simulink model "flightControlSystem"  (R2019a)
settings: Solver=ode3  StartTime=0  StopTime=TFinal  FixedStep=Ts  RelTol=1e-3  EnableMultiTasking=on
undefined symbols (not defined in the file): codertarget, Controller, DiscIntNeverNeededParam, Discrete, Estimator, g, I_pr_antiWU, I_pr_satLimitHigh, I_pr_satLimitLow, I_xy_antiWU, I_xy_satLimitHigh, I_xy_satLimitLow, I_z_antiWU, I_z_satLimitHigh, I_z_satLimitLow, init, Sensors, Time, Ts, Vehicle
libraries: simulink x35, sharedtransform x3, ctrlSharedLib x2, parrotlib x2, dspsigops x1, sharedutil x1
(part 1 of 2)

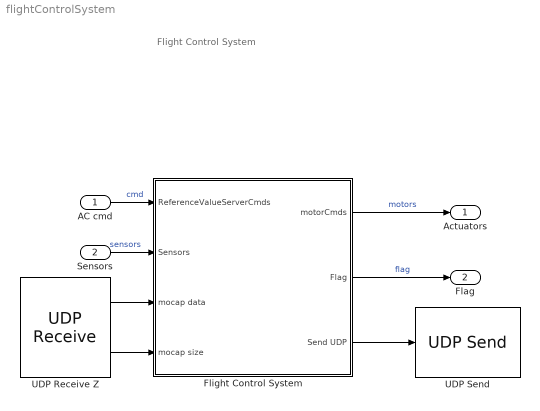
== system flightControlSystem ==
  note: Flight Control System
  AC cmd : Inport  OutDataTypeStr=Bus: CommandBus  BusOutputAsStruct=on
  Sensors : Inport  Port=2  OutDataTypeStr=Bus: SensorsBus  BusOutputAsStruct=on
  Flight Control System : Subsystem  InitFcn=codertarget.parrot.internal.fcsSubsystemCallback(gcb);  TreatAsAtomicUnit=on  SystemSampleTime=Ts
  UDP Receive Z : parrotlib/UDP Receive  localURL='0.0.0.0'  localPort=25000  remoteURL='0.0.0.0'  remotePort=-1  recvBufferSize=8192  signalDatatype=single  dims=24  isVarSize=off  showBlockingTime=off  blockingTime=0  sampletime=0.005  blockPlatform=LINUX
  UDP Send : parrotlib/UDP Send  remoteURL='192.168.3.2'  remotePort=25001  localURL='0.0.0.0'  localPortSource=Automatically determine  localPort=2048  sampletime=-1  blockPlatform=LINUX  separateLengthPort=0
  Actuators : Outport  OutDataTypeStr=single  PortDimensions=4
  Flag : Outport  Port=2  OutDataTypeStr=uint8  PortDimensions=1
  wires:
  Flight Control System/1(motorCmds) -> Actuators/1  "motors"
  Flight Control System/2(Flag) -> Flag/1  "flag"
  Flight Control System/3(Send UDP) -> UDP Send/1
  AC cmd/1 -> Flight Control System/1(ReferenceValueServerCmds)  "cmd"
  Sensors/1 -> Flight Control System/2(Sensors)  "sensors"
  UDP Receive Z/1 -> Flight Control System/3(mocap data)
  UDP Receive Z/2 -> Flight Control System/4(mocap size)

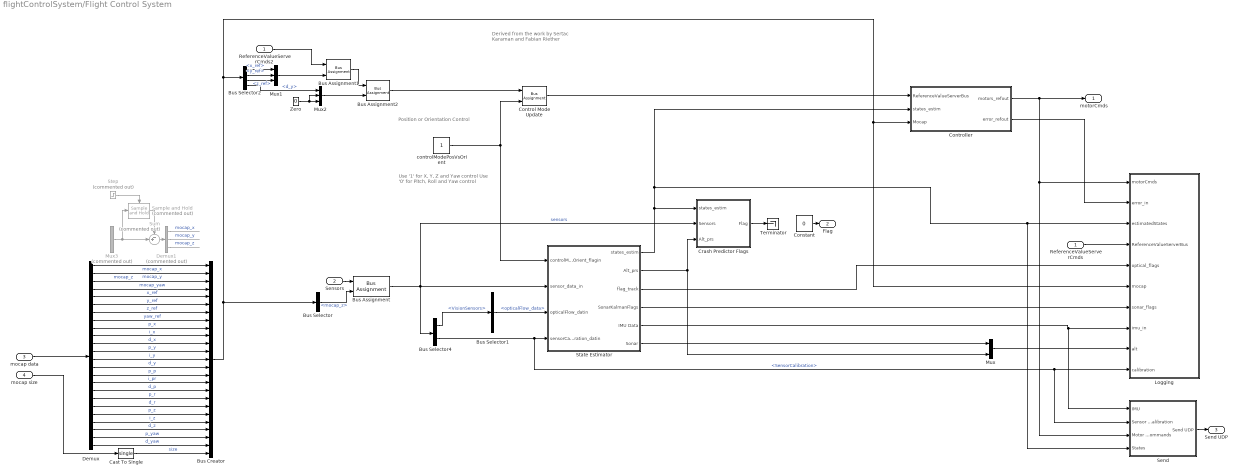
== system flightControlSystem/Flight Control System ==
  note: Use '1' for X, Y, Z and Yaw control
      | Use '0' for Pitch, Roll and Yaw control
  note: Position or Orientation Control
  note: Derived from the work by Sertac
      | Karaman and Fabian Riether
  ReferenceValueServerCmds : Inport  OutDataTypeStr=Bus: CommandBus
  Sensors : Inport  Port=2  OutDataTypeStr=Bus: SensorsBus  BusOutputAsStruct=on
  mocap data : Inport  Port=3
  mocap size : Inport  Port=4
  Bus Assignment : BusAssignment  AssignedSignals=HALSensors.HAL_ultrasound_SI.altitude
  Bus Assignment1 : BusAssignment  AssignedSignals=pos_ref
  Bus Assignment2 : BusAssignment  AssignedSignals=orient_ref
  Bus Creator : BusCreator  Inputs=25
  Bus Selector : BusSelector  OutputSignals=mocap_z
  Bus Selector1 : BusSelector  OutputSignals=opticalFlow_data
  Bus Selector2 : BusSelector  OutputSignals=x_ref,y_ref,z_ref,d_y
  Bus Selector4 : BusSelector  OutputSignals=VisionSensors,SensorCalibration
  Cast To Single : DataTypeConversion  OutDataTypeStr=single
  Constant : Constant  Value=0  OutDataTypeStr=uint8
  Control Mode Update : BusAssignment  AssignedSignals=controlModePosVSOrient
  Controller : Subsystem
  Crash Predictor Flags : Subsystem
  Demux : Demux  Outputs=24
  Demux1 : Demux  Commented=on  Outputs=3
  Logging : Subsystem  TreatAsAtomicUnit=on
  Mux : Mux  Inputs=2
  Mux1 : Mux  Inputs=3
  Mux2 : Mux  Inputs=3
  Mux3 : Mux  Commented=on  Inputs=3
  ReferenceValueServerCmds2 : InportShadow  OutDataTypeStr=Bus: CommandBus
  Sample and Hold : dspsigops/Sample and Hold  Commented=on  trig=Rising edge  initCond=0  latchinput=off
  Send : Subsystem  TreatAsAtomicUnit=on
  State Estimator : Subsystem
  Step : Step  Commented=on  Time=Ts  SampleTime=Ts
  Sum : Sum  Commented=on  Inputs=-+|
  Terminator : Terminator
  Zero : Constant  Value=0  OutDataTypeStr=single
  controlModePosVsOrient : Constant  OutDataTypeStr=boolean
  motorCmds : Outport
  Flag : Outport  Port=2
  Send UDP : Outport  Port=3
  wires:
  Bus Assignment2/1 -> Control Mode Update/1
  Bus Selector1/1 -> State Estimator/3(opticalFlow_datin)  "<opticalFlow_data>"
  Bus Selector4/2 -> Send/2(Sensor Calibration), Logging/10(calibration), State Estimator/4(sensorCalibration_datin)  "<SensorCalibration>"
  Bus Selector4/1 -> Bus Selector1/1  "<VisionSensors>"
  Controller/1(motors_refout) -> Send/3(Motor Commands), Logging/1(motorCmds), motorCmds/1
  State Estimator/1(states_estim) -> Send/4(States), Logging/3(estimatedStates), Controller/2(states_estim), Crash Predictor Flags/1(states_estim)
  State Estimator/2(Alt_prs) -> Crash Predictor Flags/3(Alt_prs), Mux/2
  Controller/2(error_refout) -> Logging/2(error_in)
  ReferenceValueServerCmds/1 -> Logging/4(ReferenceValueServerBus)
  State Estimator/3(flag_track) -> Logging/5(optical_flags)
  Control Mode Update/1 -> Controller/1(ReferenceValueServerBus)
  controlModePosVsOrient/1 -> State Estimator/1(controlModePosVSOrient_flagin), Control Mode Update/2
  State Estimator/4(SonarKalmanFlags) -> Logging/7(sonar_flags)
  State Estimator/5(IMU Data) -> Send/1(IMU), Logging/8(imu_in)
  State Estimator/6(Sonar) -> Mux/1
  Mux/1 -> Logging/9(alt)
  Crash Predictor Flags/1(Flag) -> Terminator/1
  Constant/1 -> Flag/1
  Bus Creator/1 -> Logging/6(mocap), Controller/3(Mocap), Bus Selector2/1, Bus Selector/1
  Send/1(Send UDP) -> Send UDP/1
  Cast To Single/1 -> Bus Creator/25  "size"
  Demux/9 -> Bus Creator/9  "p_x"
  Bus Selector/1 -> Bus Assignment/2  "<mocap_z>"
  Demux/5 -> Bus Creator/5  "x_ref"
  Bus Assignment/1 -> Bus Selector4/1, Crash Predictor Flags/2(Sensors), State Estimator/2(sensor_data_in)  "sensors"
  Demux/17 -> Bus Creator/17  "d_p"
  Demux/4 -> Bus Creator/4  "mocap_yaw"
  Demux/8 -> Bus Creator/8  "yaw_ref"
  Mux2/1 -> Bus Assignment2/2
  Demux/23 -> Bus Creator/23  "p_yaw"
  Demux/12 -> Bus Creator/12  "p_y"
  Demux/1 -> Bus Creator/1  "mocap_x"
  Demux/22 -> Bus Creator/22  "d_z"
  Demux/19 -> Bus Creator/19  "d_r"
  Mux1/1 -> Bus Assignment1/2
  Bus Selector2/2 -> Mux1/2  "<y_ref>"
  Bus Selector2/4 -> Mux2/1  "<d_y>"
  Demux/6 -> Bus Creator/6  "y_ref"
  Demux/18 -> Bus Creator/18  "p_r"
  mocap data/1 -> Demux/1
  Demux/2 -> Bus Creator/2  "mocap_y"
  Demux/24 -> Bus Creator/24  "d_yaw"
  Demux/14 -> Bus Creator/14  "d_y"
  Demux/13 -> Bus Creator/13  "i_y"
  Demux/21 -> Bus Creator/21  "i_z"
  Demux/20 -> Bus Creator/20  "p_z"
  mocap size/1 -> Cast To Single/1
  Demux/10 -> Bus Creator/10  "i_x"
  Demux/7 -> Bus Creator/7  "z_ref"
  Bus Assignment1/1 -> Bus Assignment2/1
  Demux/11 -> Bus Creator/11  "d_x"
  Demux/15 -> Bus Creator/15  "p_p"
  Bus Selector2/1 -> Mux1/1  "<x_ref>"
  Zero/1 -> Mux2/2, Mux2/3
  Demux/16 -> Bus Creator/16  "i_pr"
  Bus Selector2/3 -> Mux1/3  "<z_ref>"
  Demux/3 -> Bus Creator/3  "mocap_z"
  Sensors/1 -> Bus Assignment/1
  ReferenceValueServerCmds2/1 -> Bus Assignment1/1
  Step/1 -> Sample and Hold/Trigger
  Demux1/2 -> ?  "mocap_y"
  Demux1/3 -> ?  "mocap_z"
  Demux1/1 -> ?  "mocap_x"
  Sample and Hold/1 -> Sum/1
  Sum/1 -> Demux1/1
  Mux3/1 -> Sum/2, Sample and Hold/1

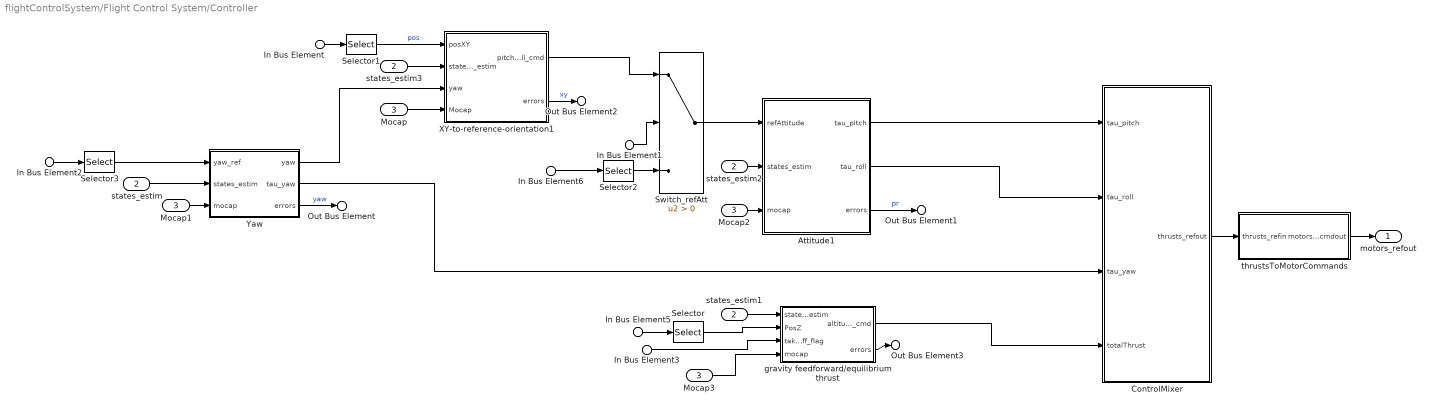
== system flightControlSystem/Flight Control System/Controller ==
  In Bus Element1 : Inport  PortName=ReferenceValueServerBus  Element=controlModePosVSOrient
  In Bus Element : Inport  PortName=ReferenceValueServerBus  Element=pos_ref
  In Bus Element5 : Inport  PortName=ReferenceValueServerBus  Element=pos_ref
  In Bus Element2 : Inport  PortName=ReferenceValueServerBus  Element=orient_ref
  In Bus Element6 : Inport  PortName=ReferenceValueServerBus  Element=orient_ref
  In Bus Element3 : Inport  PortName=ReferenceValueServerBus  Element=takeoff_flag
  states_estim : Inport  Port=2
  Mocap : Inport  Port=3
  Attitude1 : Subsystem
  ControlMixer : Subsystem
  Mocap1 : InportShadow  Port=3
  Mocap2 : InportShadow  Port=3
  Mocap3 : InportShadow  Port=3
  Selector : Selector  InputPortWidth=3  IndexOptions=Index vector (dialog)  Indices=3  OutputSizes=1
  Selector1 : Selector  InputPortWidth=3  IndexOptions=Index vector (dialog)  Indices=[1 2]  OutputSizes=1
  Selector2 : Selector  InputPortWidth=3  IndexOptions=Index vector (dialog)  Indices=[2 3]  OutputSizes=1
  Selector3 : Selector  InputPortWidth=3  IndexOptions=Index vector (dialog)  Indices=1  OutputSizes=1
  Switch_refAtt : Switch  Criteria=u2 > Threshold
  XY-to-reference-orientation1 : Subsystem
  Yaw : Subsystem
  gravity feedforward/equilibrium thrust : Subsystem
  states_estim1 : InportShadow  Port=2
  states_estim2 : InportShadow  Port=2
  states_estim3 : InportShadow  Port=2
  thrustsToMotorCommands : Subsystem
  motors_refout : Outport
  Out Bus Element : Outport  Port=2  PortName=error_refout  Element=yaw
  Out Bus Element1 : Outport  Port=2  PortName=error_refout  Element=pr
  Out Bus Element2 : Outport  Port=2  PortName=error_refout  Element=xy
  Out Bus Element3 : Outport  Port=2  PortName=error_refout  Element=z
  wires:
  thrustsToMotorCommands/1(motors_cmdout) -> motors_refout/1
  In Bus Element5/1 -> Selector/1
  Attitude1/2(tau_roll) -> ControlMixer/2(tau_roll)
  states_estim3/1 -> XY-to-reference-orientation1/2(states_estim)
  In Bus Element6/1 -> Selector2/1
  Selector3/1 -> Yaw/1(yaw_ref)
  In Bus Element/1 -> Selector1/1
  ControlMixer/1(thrusts_refout) -> thrustsToMotorCommands/1(thrusts_refin)
  Selector2/1 -> Switch_refAtt/3
  Attitude1/1(tau_pitch) -> ControlMixer/1(tau_pitch)
  gravity feedforward/equilibrium thrust/1(altitude_cmd) -> ControlMixer/4(totalThrust)
  Selector1/1 -> XY-to-reference-orientation1/1(posXY)  "pos"
  states_estim1/1 -> gravity feedforward/equilibrium thrust/1(states_estim)
  Selector/1 -> gravity feedforward/equilibrium thrust/2(PosZ)
  Yaw/1(yaw) -> XY-to-reference-orientation1/3(yaw)
  In Bus Element3/1 -> gravity feedforward/equilibrium thrust/3(takeoff_flag)
  states_estim/1 -> Yaw/2(states_estim)
  XY-to-reference-orientation1/1(pitch_roll_cmd) -> Switch_refAtt/1
  In Bus Element2/1 -> Selector3/1
  Yaw/2(tau_yaw) -> ControlMixer/3(tau_yaw)
  In Bus Element1/1 -> Switch_refAtt/2
  Switch_refAtt/1 -> Attitude1/1(refAttitude)
  states_estim2/1 -> Attitude1/2(states_estim)
  XY-to-reference-orientation1/2(errors) -> Out Bus Element2/1  "xy"
  Attitude1/3(errors) -> Out Bus Element1/1  "pr"
  gravity feedforward/equilibrium thrust/2(errors) -> Out Bus Element3/1
  Yaw/3(errors) -> Out Bus Element/1  "yaw"
  Mocap/1 -> XY-to-reference-orientation1/4(Mocap)
  Mocap1/1 -> Yaw/3(mocap)
  Mocap2/1 -> Attitude1/3(mocap)
  Mocap3/1 -> gravity feedforward/equilibrium thrust/4(mocap)

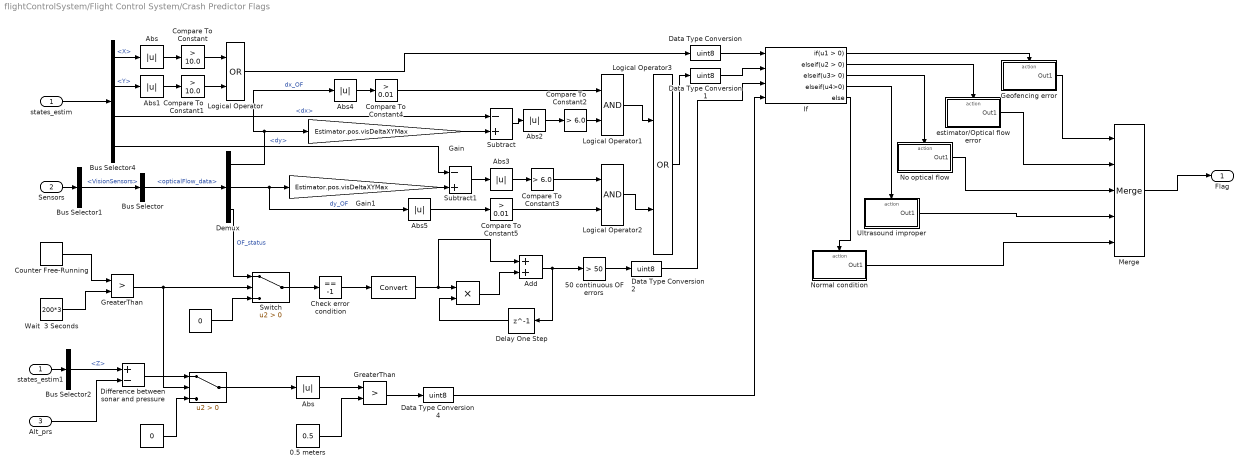
== system flightControlSystem/Flight Control System/Crash Predictor Flags ==
  states_estim : Inport
  Sensors : Inport  Port=2
  Alt_prs : Inport  Port=3
  " " : Constant  Value=0
  "  " : Product  Inputs=**
  "   " : DataTypeConversion
  "    " : Constant  Value=0  OutDataTypeStr=single
  "         " : Switch  Criteria=u2 > Threshold
  0.5 meters : Constant  Value=0.5
  "50 continuous OF errors " : simulink/Logic and Bit Operations/Compare To Constant  relop=>  const=50  OutDataTypeStr=boolean
  Abs{,1..5} (6 alike) : Abs
  "Abs  " : Abs
  Add : Sum
  Bus Selector : BusSelector  OutputSignals=opticalFlow_data
  Bus Selector1 : BusSelector  OutputSignals=VisionSensors
  Bus Selector2 : BusSelector  OutputSignals=Z
  Bus Selector4 : BusSelector  OutputSignals=X,Y,dx,dy
  Check error condition : simulink/Logic and Bit Operations/Compare To Constant  relop===  const=-1  OutDataTypeStr=boolean
  Compare To Constant : simulink/Logic and Bit Operations/Compare To Constant  relop=>  const=10.0  OutDataTypeStr=boolean
  Compare To Constant1 : simulink/Logic and Bit Operations/Compare To Constant  relop=>  const=10.0  OutDataTypeStr=boolean
  Compare To Constant2 : simulink/Logic and Bit Operations/Compare To Constant  relop=>  const=6.0  OutDataTypeStr=boolean
  Compare To Constant3 : simulink/Logic and Bit Operations/Compare To Constant  relop=>  const=6.0  OutDataTypeStr=boolean
  Compare To Constant4 : simulink/Logic and Bit Operations/Compare To Constant  relop=>  const=0.01  OutDataTypeStr=boolean
  Compare To Constant5 : simulink/Logic and Bit Operations/Compare To Constant  relop=>  const=0.01  OutDataTypeStr=boolean
  Counter Free-Running : simulink/Sources/Counter Free-Running  NumBits=32  tsamp=-1
  Data Type Conversion{,1..2,4} (4 alike) : DataTypeConversion  OutDataTypeStr=uint8  RndMeth=Nearest
  Delay One Step : Delay  DelayLength=1
  Demux : Demux  Outputs=3
  Difference between sonar and pressure : Sum  Inputs=+-
  Gain : Gain  Gain=Estimator.pos.visDeltaXYMax
  Gain1 : Gain  Gain=Estimator.pos.visDeltaXYMax
  Geofencing error : Subsystem  TreatAsAtomicUnit=on
  GreaterThan : RelationalOperator  Operator=>  OutDataTypeStr=boolean  RndMeth=Simplest
  "GreaterThan  " : RelationalOperator  Operator=>  OutDataTypeStr=boolean  RndMeth=Simplest
  If : If  NumInputs=4  ElseIfExpressions=u2 > 0, u3> 0,u4>0
  Logical Operator : Logic  Operator=OR  AllPortsSameDT=off
  Logical Operator1 : Logic  AllPortsSameDT=off  OutDataTypeStr=boolean
  Logical Operator2 : Logic  AllPortsSameDT=off  OutDataTypeStr=boolean
  Logical Operator3 : Logic  Operator=OR  AllPortsSameDT=off
  Merge : Merge  Inputs=5  InitialOutput=0
  "No optical flow " : Subsystem  TreatAsAtomicUnit=on
  Normal condition : Subsystem  TreatAsAtomicUnit=on
  Subtract : Sum  Inputs=-+
  Subtract1 : Sum  Inputs=-+
  Switch : Switch  Criteria=u2 > Threshold
  Ultrasound improper : Subsystem  TreatAsAtomicUnit=on
  Wait  3 Seconds : Constant  Value=200*3
  estimator/Optical flow error : Subsystem  TreatAsAtomicUnit=on
  states_estim1 : InportShadow
  Flag : Outport
  wires:
  Bus Selector4/1 -> Abs/1  "<X>"
  states_estim/1 -> Bus Selector4/1
  Bus Selector4/2 -> Abs1/1  "<Y>"
  Compare To Constant/1 -> Logical Operator/1
  Compare To Constant1/1 -> Logical Operator/2
  Abs/1 -> Compare To Constant/1
  Abs1/1 -> Compare To Constant1/1
  Logical Operator/1 -> Data Type Conversion/1
  Bus Selector/1 -> Demux/1  "<opticalFlow_data>"
  Demux/1 -> Abs4/1, Gain/1  "dx_OF"
  Demux/2 -> Gain1/1, Abs5/1  "dy_OF"
  Bus Selector4/3 -> Subtract/1  "<dx>"
  Subtract/1 -> Abs2/1
  Subtract1/1 -> Abs3/1
  Abs2/1 -> Compare To Constant2/1
  Abs3/1 -> Compare To Constant3/1
  Compare To Constant5/1 -> Logical Operator2/2
  Abs4/1 -> Compare To Constant4/1
  Abs5/1 -> Compare To Constant5/1
  Compare To Constant3/1 -> Logical Operator2/1
  Logical Operator1/1 -> Logical Operator3/1
  Logical Operator2/1 -> Logical Operator3/2
  Logical Operator3/1 -> Data Type Conversion1/1
  Gain/1 -> Subtract/2
  Bus Selector4/4 -> Subtract1/1  "<dy>"
  Gain1/1 -> Subtract1/2
  Compare To Constant4/1 -> Logical Operator1/1
  Compare To Constant2/1 -> Logical Operator1/2
  Sensors/1 -> Bus Selector1/1
  Bus Selector1/1 -> Bus Selector/1  "<VisionSensors>"
  Merge/1 -> Flag/1
  If/1 -> Geofencing error/Action
  If/2 -> estimator/Optical flow error/Action
  If/5 -> Normal condition/Action
  Geofencing error/1(Out1) -> Merge/1
  estimator/Optical flow error/1(Out1) -> Merge/2
  Normal condition/1(Out1) -> Merge/5
  Data Type Conversion/1 -> If/1
  Data Type Conversion1/1 -> If/2
  Check error condition/1 -> "   "/1
  Demux/3 -> Switch/1  "OF_status"
  Delay One Step/1 -> "  "/2
  Add/1 -> Delay One Step/1, "50 continuous OF errors "/1
  "  "/1 -> Add/2
  "50 continuous OF errors "/1 -> Data Type Conversion2/1
  Data Type Conversion2/1 -> If/3
  "No optical flow "/1(Out1) -> Merge/3
  If/3 -> "No optical flow "/Action
  "   "/1 -> Add/1, "  "/1
  Counter Free-Running/1 -> GreaterThan/1
  Wait  3 Seconds/1 -> GreaterThan/2
  Switch/1 -> Check error condition/1
  " "/1 -> Switch/3
  "    "/1 -> "         "/3
  Difference between sonar and pressure/1 -> "         "/1
  Bus Selector2/1 -> Difference between sonar and pressure/1  "<Z>"
  GreaterThan/1 -> Switch/2, "         "/2
  "         "/1 -> "Abs  "/1
  "Abs  "/1 -> "GreaterThan  "/1
  0.5 meters/1 -> "GreaterThan  "/2
  Alt_prs/1 -> Difference between sonar and pressure/2
  "GreaterThan  "/1 -> Data Type Conversion4/1
  states_estim1/1 -> Bus Selector2/1
  Data Type Conversion4/1 -> If/4
  Ultrasound improper/1(Out1) -> Merge/4
  If/4 -> Ultrasound improper/Action

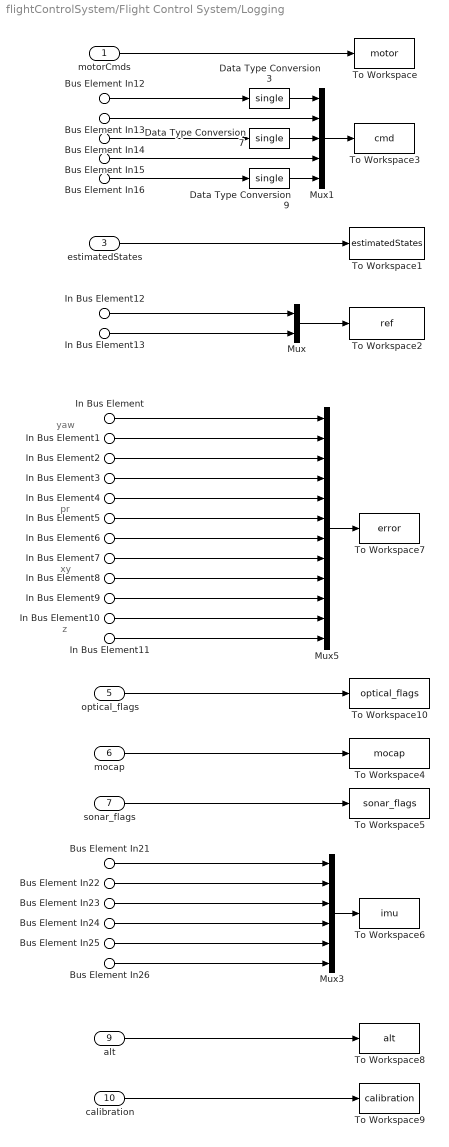
== system flightControlSystem/Flight Control System/Logging ==
  note: yaw
  note: pr
  note: xy
  note: z
  motorCmds : Inport
  In Bus Element : Inport  Port=2  PortName=error_in  Element=yaw.p
  In Bus Element1 : Inport  Port=2  PortName=error_in  Element=yaw.i
  In Bus Element2 : Inport  Port=2  PortName=error_in  Element=yaw.d
  In Bus Element3 : Inport  Port=2  PortName=error_in  Element=pr.p
  In Bus Element4 : Inport  Port=2  PortName=error_in  Element=pr.i
  In Bus Element5 : Inport  Port=2  PortName=error_in  Element=pr.d
  In Bus Element6 : Inport  Port=2  PortName=error_in  Element=xy.p
  In Bus Element7 : Inport  Port=2  PortName=error_in  Element=xy.i
  In Bus Element8 : Inport  Port=2  PortName=error_in  Element=xy.d
  In Bus Element9 : Inport  Port=2  PortName=error_in  Element=z.p
  In Bus Element10 : Inport  Port=2  PortName=error_in  Element=z.i
  In Bus Element11 : Inport  Port=2  PortName=error_in  Element=z.d
  estimatedStates : Inport  Port=3
  Bus Element In12 : Inport  Port=4  PortName=ReferenceValueServerBus  Element=controlModePosVSOrient
  Bus Element In13 : Inport  Port=4  PortName=ReferenceValueServerBus  Element=pos_ref
  In Bus Element12 : Inport  Port=4  PortName=ReferenceValueServerBus  Element=pos_ref
  Bus Element In14 : Inport  Port=4  PortName=ReferenceValueServerBus  Element=takeoff_flag
  Bus Element In15 : Inport  Port=4  PortName=ReferenceValueServerBus  Element=orient_ref
  In Bus Element13 : Inport  Port=4  PortName=ReferenceValueServerBus  Element=orient_ref
  Bus Element In16 : Inport  Port=4  PortName=ReferenceValueServerBus  Element=live_time_ticks
  optical_flags : Inport  Port=5
  mocap : Inport  Port=6
  sonar_flags : Inport  Port=7
  Bus Element In21 : Inport  Port=8  PortName=imu_in  Element=ddx
  Bus Element In22 : Inport  Port=8  PortName=imu_in  Element=ddy
  Bus Element In23 : Inport  Port=8  PortName=imu_in  Element=ddz
  Bus Element In24 : Inport  Port=8  PortName=imu_in  Element=p
  Bus Element In25 : Inport  Port=8  PortName=imu_in  Element=q
  Bus Element In26 : Inport  Port=8  PortName=imu_in  Element=r
  alt : Inport  Port=9
  calibration : Inport  Port=10
  Data Type Conversion3 : DataTypeConversion  OutDataTypeStr=single
  Data Type Conversion7 : DataTypeConversion  OutDataTypeStr=single
  Data Type Conversion9 : DataTypeConversion  OutDataTypeStr=single
  Mux : Mux  Inputs=2
  Mux1 : Mux  Inputs=5
  Mux3 : Mux  Inputs=6
  Mux5 : Mux  Inputs=12
  To Workspace : ToWorkspace  VariableName=motor  SaveFormat=Structure With Time  SampleTime=-1
  To Workspace1 : ToWorkspace  VariableName=estimatedStates  SaveFormat=Structure With Time  SampleTime=-1
  To Workspace10 : ToWorkspace  VariableName=optical_flags  SaveFormat=Structure With Time  SampleTime=-1
  To Workspace2 : ToWorkspace  VariableName=ref  SaveFormat=Structure With Time  SampleTime=-1
  To Workspace3 : ToWorkspace  VariableName=cmd  SaveFormat=Structure With Time  SampleTime=-1
  To Workspace4 : ToWorkspace  VariableName=mocap  SaveFormat=Structure With Time  SampleTime=-1
  To Workspace5 : ToWorkspace  VariableName=sonar_flags  SaveFormat=Structure With Time  SampleTime=-1
  To Workspace6 : ToWorkspace  VariableName=imu  SaveFormat=Structure With Time  SampleTime=-1
  To Workspace7 : ToWorkspace  VariableName=error  SaveFormat=Structure With Time  SampleTime=-1
  To Workspace8 : ToWorkspace  VariableName=alt  SaveFormat=Structure With Time  SampleTime=-1
  To Workspace9 : ToWorkspace  VariableName=calibration  SaveFormat=Structure With Time  SampleTime=-1
  wires:
  Bus Element In12/1 -> Data Type Conversion3/1
  Bus Element In14/1 -> Data Type Conversion7/1
  Bus Element In16/1 -> Data Type Conversion9/1
  motorCmds/1 -> To Workspace/1
  Mux1/1 -> To Workspace3/1
  Data Type Conversion3/1 -> Mux1/1
  Bus Element In13/1 -> Mux1/2
  Data Type Conversion7/1 -> Mux1/3
  Bus Element In15/1 -> Mux1/4
  Data Type Conversion9/1 -> Mux1/5
  In Bus Element/1 -> Mux5/1
  In Bus Element1/1 -> Mux5/2
  In Bus Element2/1 -> Mux5/3
  In Bus Element3/1 -> Mux5/4
  In Bus Element4/1 -> Mux5/5
  In Bus Element5/1 -> Mux5/6
  In Bus Element11/1 -> Mux5/12
  In Bus Element10/1 -> Mux5/11
  In Bus Element9/1 -> Mux5/10
  In Bus Element8/1 -> Mux5/9
  In Bus Element7/1 -> Mux5/8
  In Bus Element6/1 -> Mux5/7
  Mux5/1 -> To Workspace7/1
  optical_flags/1 -> To Workspace10/1
  estimatedStates/1 -> To Workspace1/1
  In Bus Element13/1 -> Mux/2
  Mux/1 -> To Workspace2/1
  In Bus Element12/1 -> Mux/1
  mocap/1 -> To Workspace4/1
  sonar_flags/1 -> To Workspace5/1
  Bus Element In25/1 -> Mux3/5
  Bus Element In22/1 -> Mux3/2
  Bus Element In21/1 -> Mux3/1
  Bus Element In23/1 -> Mux3/3
  Mux3/1 -> To Workspace6/1
  Bus Element In26/1 -> Mux3/6
  Bus Element In24/1 -> Mux3/4
  alt/1 -> To Workspace8/1
  calibration/1 -> To Workspace9/1

== system flightControlSystem/Flight Control System/Send ==
  IMU : Inport
  Sensor Calibration : Inport  Port=2
  Motor Commands : Inport  Port=3
  States : Inport  Port=4
  Bus Selector : BusSelector  OutputSignals=ddx,ddy,ddz
  Bus Selector3 : BusSelector  OutputSignals=yaw,pitch,roll,dx,dy,dz,p,q,r
  Constant : Constant  OutDataTypeStr=single
  Demux : Demux
  Demux1 : Demux  Outputs=8
  Mux : Mux  Inputs=5
  Mux2 : Mux  Inputs=20
  Terminator : Terminator
  Send UDP : Outport
  wires:
  IMU/1 -> Bus Selector/1
  Sensor Calibration/1 -> Demux1/1
  Motor Commands/1 -> Demux/1
  States/1 -> Bus Selector3/1
  Bus Selector/1 -> Mux2/2  "<ddx>"
  Bus Selector/2 -> Mux2/3  "<ddy>"
  Bus Selector/3 -> Mux2/4  "<ddz>"
  Demux1/1 -> Mux2/5
  Demux1/2 -> Mux2/6
  Demux1/3 -> Mux2/7
  Constant/1 -> Mux2/1
  Mux2/1 -> Send UDP/1
  Demux1/6 -> Mux/3
  Demux1/4 -> Mux/1
  Demux1/5 -> Mux/2
  Demux1/7 -> Mux/4
  Demux1/8 -> Mux/5
  Mux/1 -> Terminator/1
  Demux/1 -> Mux2/8
  Demux/2 -> Mux2/9
  Demux/3 -> Mux2/10
  Demux/4 -> Mux2/11
  Bus Selector3/1 -> Mux2/12  "<yaw>"
  Bus Selector3/2 -> Mux2/13  "<pitch>"
  Bus Selector3/3 -> Mux2/14  "<roll>"
  Bus Selector3/4 -> Mux2/15  "<dx>"
  Bus Selector3/5 -> Mux2/16  "<dy>"
  Bus Selector3/6 -> Mux2/17  "<dz>"
  Bus Selector3/7 -> Mux2/18  "<p>"
  Bus Selector3/8 -> Mux2/19  "<q>"
  Bus Selector3/9 -> Mux2/20  "<r>"

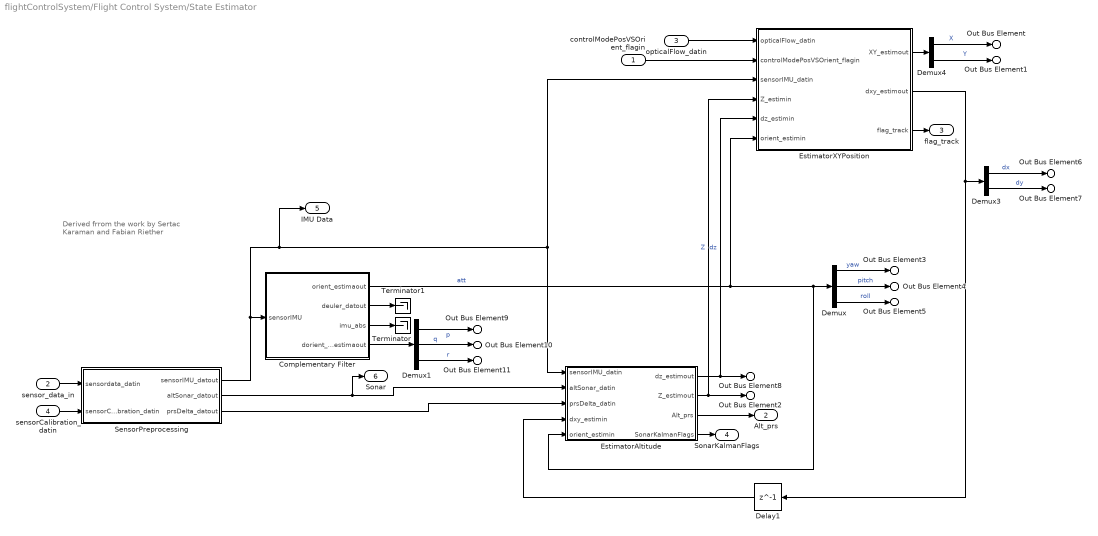
== system flightControlSystem/Flight Control System/State Estimator ==
  note: Derived frrom the work by Sertac
      | Karaman and Fabian Riether
  controlModePosVSOrient_flagin : Inport  OutDataTypeStr=boolean
  sensor_data_in : Inport  Port=2
  opticalFlow_datin : Inport  Port=3
  sensorCalibration_datin : Inport  Port=4
  Complementary Filter : Subsystem
  Delay1 : Delay  DelayLength=1  InitialCondition=0
  Demux : Demux  Outputs=3
  Demux1 : Demux  Outputs=3
  Demux3 : Demux  Outputs=2
  Demux4 : Demux  Outputs=2
  EstimatorAltitude : Subsystem
  EstimatorXYPosition : Subsystem
  SensorPreprocessing : Subsystem
  Terminator : Terminator
  Terminator1 : Terminator
  Out Bus Element : Outport  PortName=states_estim  Element=X
  Out Bus Element1 : Outport  PortName=states_estim  Element=Y
  Out Bus Element2 : Outport  PortName=states_estim  Element=Z
  Out Bus Element3 : Outport  PortName=states_estim  Element=yaw
  Out Bus Element4 : Outport  PortName=states_estim  Element=pitch
  Out Bus Element5 : Outport  PortName=states_estim  Element=roll
  Out Bus Element6 : Outport  PortName=states_estim  Element=dx
  Out Bus Element7 : Outport  PortName=states_estim  Element=dy
  Out Bus Element8 : Outport  PortName=states_estim  Element=dz
  Out Bus Element9 : Outport  PortName=states_estim  Element=p
  Out Bus Element10 : Outport  PortName=states_estim  Element=q
  Out Bus Element11 : Outport  PortName=states_estim  Element=r
  Alt_prs : Outport  Port=2
  flag_track : Outport  Port=3
  SonarKalmanFlags : Outport  Port=4
  IMU Data : Outport  Port=5
  Sonar : Outport  Port=6
  wires:
  EstimatorXYPosition/2(dxy_estimout) -> Delay1/1, Demux3/1
  Demux1/3 -> Out Bus Element11/1  "r"
  Demux/3 -> Out Bus Element5/1  "roll"
  Demux4/2 -> Out Bus Element1/1  "Y"
  EstimatorXYPosition/1(XY_estimout) -> Demux4/1
  Complementary Filter/2(deuler_datout) -> Terminator1/1
  Complementary Filter/4(dorient_estimaout) -> Demux1/1
  sensor_data_in/1 -> SensorPreprocessing/1(sensordata_datin)
  opticalFlow_datin/1 -> EstimatorXYPosition/1(opticalFlow_datin)
  Demux4/1 -> Out Bus Element/1  "X"
  SensorPreprocessing/1(sensorIMU_datout) -> IMU Data/1, EstimatorAltitude/1(sensorIMU_datin), EstimatorXYPosition/3(sensorIMU_datin), Complementary Filter/1(sensorIMU)
  SensorPreprocessing/3(prsDelta_datout) -> EstimatorAltitude/3(prsDelta_datin)
  Demux3/2 -> Out Bus Element7/1  "dy"
  EstimatorAltitude/1(dz_estimout) -> EstimatorXYPosition/5(dz_estimin), Out Bus Element8/1  "dz"
  EstimatorAltitude/2(Z_estimout) -> Out Bus Element2/1, EstimatorXYPosition/4(Z_estimin)  "Z"
  Demux1/1 -> Out Bus Element9/1  "p"
  Demux3/1 -> Out Bus Element6/1  "dx"
  Complementary Filter/3(imu_abs) -> Terminator/1
  Demux/2 -> Out Bus Element4/1  "pitch"
  controlModePosVSOrient_flagin/1 -> EstimatorXYPosition/2(controlModePosVSOrient_flagin)
  Complementary Filter/1(orient_estimaout) -> EstimatorAltitude/5(orient_estimin), Demux/1, EstimatorXYPosition/6(orient_estimin)  "att"
  Demux/1 -> Out Bus Element3/1  "yaw"
  Delay1/1 -> EstimatorAltitude/4(dxy_estimin)
  Demux1/2 -> Out Bus Element10/1  "q"
  sensorCalibration_datin/1 -> SensorPreprocessing/2(sensorCalibration_datin)
  EstimatorAltitude/3(Alt_prs) -> Alt_prs/1
  EstimatorXYPosition/3(flag_track) -> flag_track/1
  EstimatorAltitude/4(SonarKalmanFlags) -> SonarKalmanFlags/1
  SensorPreprocessing/2(altSonar_datout) -> Sonar/1, EstimatorAltitude/2(altSonar_datin)

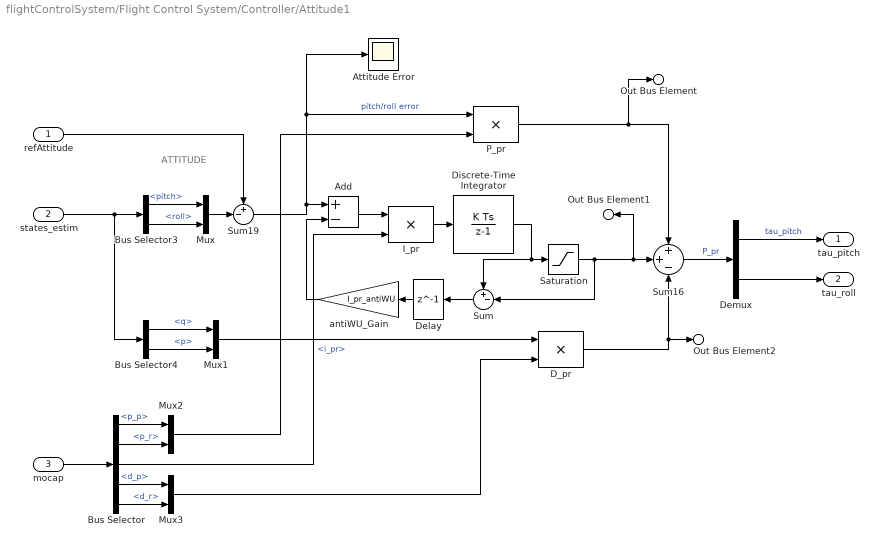
== system flightControlSystem/Flight Control System/Controller/Attitude1 ==
  note: ATTITUDE
  refAttitude : Inport
  states_estim : Inport  Port=2
  mocap : Inport  Port=3
  Add : Sum  Inputs=+-
  Attitude Error : Scope
  Bus Selector : BusSelector  OutputSignals=p_p,p_r,i_pr,d_p,d_r
  Bus Selector3 : BusSelector  OutputSignals=pitch,roll
  Bus Selector4 : BusSelector  OutputSignals=q,p
  D_pr : Product
  Delay : Delay  DelayLength=1  InitialCondition=0
  Demux : Demux  Outputs=2
  Discrete-Time Integrator : DiscreteIntegrator  gainval=1  SampleTime=Ts  UpperSaturationLimit=I_pr_satLimitHigh  LowerSaturationLimit=I_pr_satLimitLow  ICPrevOutput=DiscIntNeverNeededParam  ICPrevScaledInput=DiscIntNeverNeededParam
  I_pr : Product
  Mux{,1..3} (4 alike) : Mux  Inputs=2
  P_pr : Product
  Saturation : Saturate  UpperLimit=I_pr_satLimitHigh  LowerLimit=I_pr_satLimitLow
  Sum : Sum  Inputs=+-|
  Sum16 : Sum  Inputs=++-  AccumDataTypeStr=single  OutDataTypeStr=single  SaturateOnIntegerOverflow=on
  Sum19 : Sum  Inputs=+-|
  antiWU_Gain : Gain  Gain=I_pr_antiWU
  tau_pitch : Outport
  tau_roll : Outport  Port=2
  Out Bus Element : Outport  Port=3  PortName=errors  Element=p
  Out Bus Element1 : Outport  Port=3  PortName=errors  Element=i
  Out Bus Element2 : Outport  Port=3  PortName=errors  Element=d
  wires:
  Sum16/1 -> Demux/1  "P_pr"
  antiWU_Gain/1 -> Add/2
  Bus Selector3/1 -> Mux/1  "<pitch>"
  Bus Selector4/1 -> Mux1/1  "<q>"
  P_pr/1 -> Out Bus Element/1, Sum16/1
  Saturation/1 -> Sum/2, Out Bus Element1/1, Sum16/2
  Sum19/1 -> Add/1, P_pr/1, Attitude Error/1  "pitch/roll error"
  Delay/1 -> antiWU_Gain/1
  Demux/1 -> tau_pitch/1  "tau_pitch"
  Demux/2 -> tau_roll/1
  states_estim/1 -> Bus Selector3/1, Bus Selector4/1
  refAttitude/1 -> Sum19/1
  Mux/1 -> Sum19/2
  Bus Selector3/2 -> Mux/2  "<roll>"
  Mux1/1 -> D_pr/1
  Bus Selector4/2 -> Mux1/2  "<p>"
  D_pr/1 -> Out Bus Element2/1, Sum16/3
  Sum/1 -> Delay/1
  mocap/1 -> Bus Selector/1
  I_pr/1 -> Discrete-Time Integrator/1
  Add/1 -> I_pr/1
  Bus Selector/1 -> Mux2/1  "<p_p>"
  Bus Selector/2 -> Mux2/2  "<p_r>"
  Bus Selector/4 -> Mux3/1  "<d_p>"
  Bus Selector/5 -> Mux3/2  "<d_r>"
  Mux2/1 -> P_pr/2
  Mux3/1 -> D_pr/2
  Bus Selector/3 -> I_pr/2  "<i_pr>"
  Discrete-Time Integrator/1 -> Sum/1, Saturation/1

== system flightControlSystem/Flight Control System/Controller/ControlMixer ==
  tau_pitch : Inport
  tau_roll : Inport  Port=2
  tau_yaw : Inport  Port=3
  totalThrust : Inport  Port=4
  Mux2 : Mux
  Product : Product  Multiplication=Matrix(*)  RndMeth=Zero
  TorqueTotalThrustToThrustPerMotor : Constant  Value=Controller.Q2Ts  OutDataTypeStr=single
  thrusts_refout : Outport
  wires:
  Product/1 -> thrusts_refout/1
  tau_roll/1 -> Mux2/4
  tau_pitch/1 -> Mux2/3
  tau_yaw/1 -> Mux2/2
  totalThrust/1 -> Mux2/1
  TorqueTotalThrustToThrustPerMotor/1 -> Product/1
  Mux2/1 -> Product/2

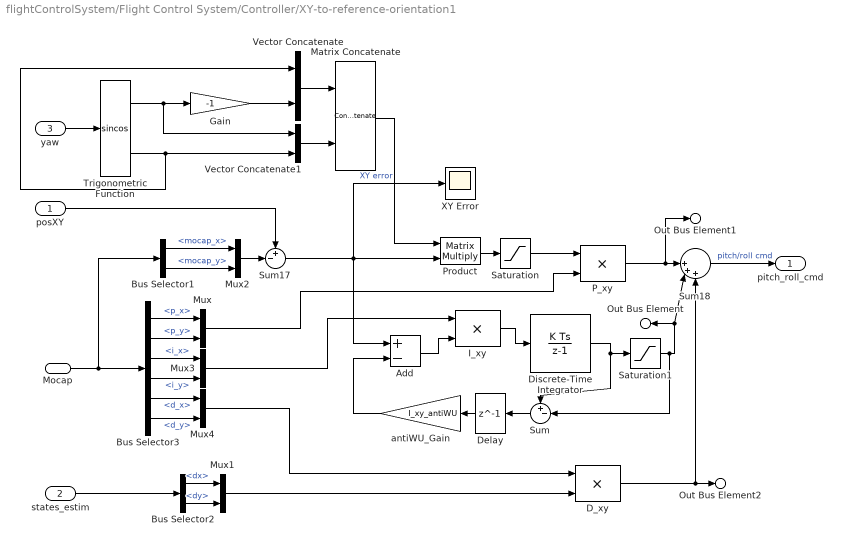
== system flightControlSystem/Flight Control System/Controller/XY-to-reference-orientation1 ==
  posXY : Inport
  states_estim : Inport  Port=2
  yaw : Inport  Port=3
  Mocap : Inport  Port=4
  Add : Sum  Inputs=+-
  Bus Selector1 : BusSelector  OutputSignals=mocap_x,mocap_y
  Bus Selector2 : BusSelector  OutputSignals=dx,dy
  Bus Selector3 : BusSelector  OutputSignals=p_x,p_y,i_x,i_y,d_x,d_y
  D_xy : Product
  Delay : Delay  DelayLength=1  InitialCondition=0
  Discrete-Time Integrator : DiscreteIntegrator  gainval=1  SampleTime=Ts  UpperSaturationLimit=I_xy_satLimitHigh  LowerSaturationLimit=I_xy_satLimitLow  ICPrevOutput=DiscIntNeverNeededParam  ICPrevScaledInput=DiscIntNeverNeededParam
  Gain : Gain  Gain=-1
  I_xy : Product
  Matrix Concatenate : Concatenate  Mode=Multidimensional array  ConcatenateDimension=2
  Mux{,1..4} (5 alike) : Mux  Inputs=2
  P_xy : Product
  Product : Product  Multiplication=Matrix(*)  OutDataTypeStr=single  RndMeth=Zero
  Saturation : Saturate  UpperLimit=3  LowerLimit=-3  OutDataTypeStr=single
  Saturation1 : Saturate  UpperLimit=I_xy_satLimitHigh  LowerLimit=I_xy_satLimitLow
  Sum : Sum  Inputs=+-|
  Sum17 : Sum  Inputs=+-|  AccumDataTypeStr=single
  Sum18 : Sum  Inputs=||+++  AccumDataTypeStr=single  OutDataTypeStr=single  SaturateOnIntegerOverflow=on
  Trigonometric Function : Trigonometry  Operator=sincos
  Vector Concatenate : Concatenate
  Vector Concatenate1 : Concatenate
  XY Error : Scope
  antiWU_Gain : Gain  Gain=I_xy_antiWU
  pitch_roll_cmd : Outport
  Out Bus Element1 : Outport  Port=2  PortName=errors  Element=p
  Out Bus Element : Outport  Port=2  PortName=errors  Element=i
  Out Bus Element2 : Outport  Port=2  PortName=errors  Element=d
  wires:
  yaw/1 -> Trigonometric Function/1
  P_xy/1 -> Out Bus Element1/1, Sum18/1
  Sum17/1 -> XY Error/1, Add/1, Product/2  "XY error"
  Bus Selector2/1 -> Mux1/1  "<dx>"
  states_estim/1 -> Bus Selector2/1
  Sum18/1 -> pitch_roll_cmd/1  "pitch/roll cmd"
  D_xy/1 -> Out Bus Element2/1, Sum18/3
  Product/1 -> Saturation/1
  Trigonometric Function/1 -> Gain/1, Vector Concatenate1/1
  Trigonometric Function/2 -> Vector Concatenate1/2, Vector Concatenate/1
  Gain/1 -> Vector Concatenate/2
  Vector Concatenate/1 -> Matrix Concatenate/1
  Vector Concatenate1/1 -> Matrix Concatenate/2
  Matrix Concatenate/1 -> Product/1
  Mux1/1 -> D_xy/2
  Bus Selector2/2 -> Mux1/2  "<dy>"
  antiWU_Gain/1 -> Add/2
  Delay/1 -> antiWU_Gain/1
  posXY/1 -> Sum17/1
  Saturation1/1 -> Sum/2, Sum18/2, Out Bus Element/1
  Sum/1 -> Delay/1
  Add/1 -> I_xy/2
  I_xy/1 -> Discrete-Time Integrator/1
  Mux2/1 -> Sum17/2
  Bus Selector1/2 -> Mux2/2  "<mocap_y>"
  Bus Selector1/1 -> Mux2/1  "<mocap_x>"
  Mocap/1 -> Bus Selector1/1, Bus Selector3/1
  Mux4/1 -> D_xy/1
  Mux/1 -> P_xy/2
  Saturation/1 -> P_xy/1
  Mux3/1 -> I_xy/1
  Bus Selector3/1 -> Mux/1  "<p_x>"
  Bus Selector3/2 -> Mux/2  "<p_y>"
  Bus Selector3/3 -> Mux3/1  "<i_x>"
  Bus Selector3/4 -> Mux3/2  "<i_y>"
  Bus Selector3/5 -> Mux4/1  "<d_x>"
  Bus Selector3/6 -> Mux4/2  "<d_y>"
  Discrete-Time Integrator/1 -> Sum/1, Saturation1/1

== system flightControlSystem/Flight Control System/Controller/Yaw ==
  yaw_ref : Inport
  states_estim : Inport  Port=2
  mocap : Inport  Port=3
  Bus Selector : BusSelector  OutputSignals=p_yaw,d_yaw
  Bus Selector5 : BusSelector  OutputSignals=yaw,r
  Constant : Constant  Value=0  OutDataTypeStr=single
  D_yaw : Product
  P_yaw : Product
  Sum1 : Sum  Inputs=+-|  AccumDataTypeStr=single  OutDataTypeStr=single  SaturateOnIntegerOverflow=on
  Sum2 : Sum  Inputs=|+-
  yaw : Outport
  tau_yaw : Outport  Port=2
  Out Bus Element : Outport  Port=3  PortName=errors  Element=p
  Out Bus Element2 : Outport  Port=3  PortName=errors  Element=i
  Out Bus Element1 : Outport  Port=3  PortName=errors  Element=d
  wires:
  D_yaw/1 -> Sum2/2, Out Bus Element1/1
  P_yaw/1 -> Out Bus Element/1, Sum2/1
  Bus Selector5/2 -> D_yaw/1  "<r>"
  Sum1/1 -> P_yaw/1
  states_estim/1 -> Bus Selector5/1
  Sum2/1 -> tau_yaw/1
  Bus Selector5/1 -> Sum1/2, yaw/1  "<yaw>"
  yaw_ref/1 -> Sum1/1
  Constant/1 -> Out Bus Element2/1
  mocap/1 -> Bus Selector/1
  Bus Selector/1 -> P_yaw/2  "<p_yaw>"
  Bus Selector/2 -> D_yaw/2  "<d_yaw>"

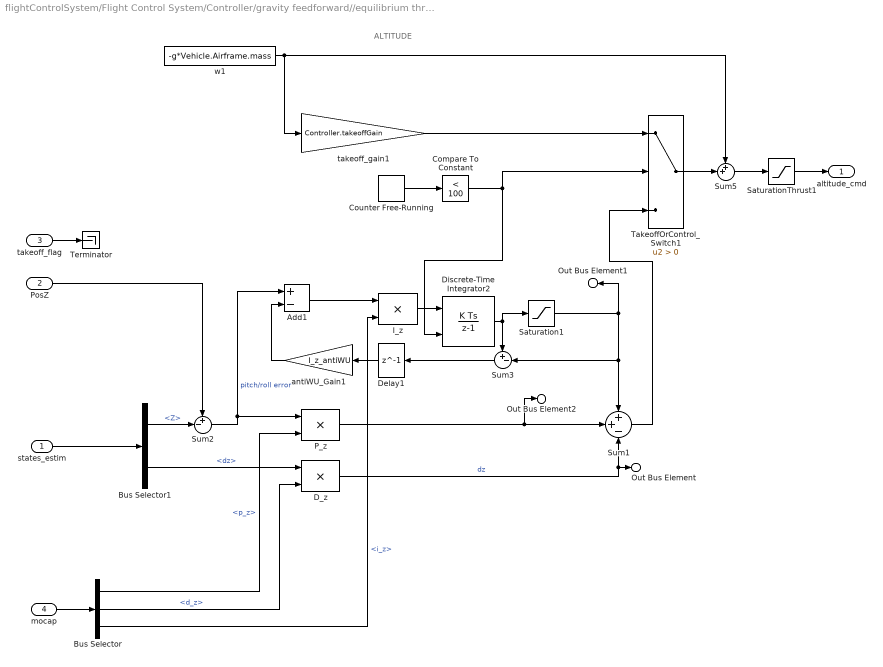
== system flightControlSystem/Flight Control System/Controller/gravity feedforward//equilibrium thrust ==
  note: ALTITUDE
  states_estim : Inport
  PosZ : Inport  Port=2
  takeoff_flag : Inport  Port=3
  mocap : Inport  Port=4
  Add1 : Sum  Inputs=+-
  Bus Selector : BusSelector  OutputSignals=p_z,d_z,i_z
  Bus Selector1 : BusSelector  OutputSignals=Z,dz
  Compare To Constant : simulink/Logic and Bit Operations/Compare To Constant  relop=<  const=100  OutDataTypeStr=boolean
  Counter Free-Running : simulink/Sources/Counter Free-Running  NumBits=16  tsamp=-1
  D_z : Product
  Delay1 : Delay  DelayLength=1  InitialCondition=0
  Discrete-Time Integrator2 : DiscreteIntegrator  gainval=1  ExternalReset=falling  SampleTime=Ts  UpperSaturationLimit=I_z_satLimitHigh  LowerSaturationLimit=I_z_satLimitLow  ICPrevOutput=DiscIntNeverNeededParam  ICPrevScaledInput=DiscIntNeverNeededParam
  I_z : Product
  P_z : Product
  Saturation1 : Saturate  UpperLimit=I_z_satLimitHigh  LowerLimit=I_z_satLimitLow
  SaturationThrust1 : Saturate  UpperLimit=4*Controller.totalThrustMaxRelative*Controller.motorsThrustPerMotorMax  LowerLimit=-4*Controller.totalThrustMaxRelative*Controller.motorsThrustPerMotorMax  OutDataTypeStr=single
  Sum1 : Sum  Inputs=++-  AccumDataTypeStr=single  OutDataTypeStr=single  SaturateOnIntegerOverflow=on
  Sum2 : Sum  Inputs=+-|  AccumDataTypeStr=single  OutDataTypeStr=single  SaturateOnIntegerOverflow=on
  Sum3 : Sum  Inputs=+-|
  Sum5 : Sum  Inputs=++|  AccumDataTypeStr=single  OutDataTypeStr=single  SaturateOnIntegerOverflow=on
  TakeoffOrControl_Switch1 : Switch  Criteria=u2 > Threshold
  Terminator : Terminator
  antiWU_Gain1 : Gain  Gain=I_z_antiWU
  takeoff_gain1 : Gain  Gain=Controller.takeoffGain  ParamDataTypeStr=single  OutDataTypeStr=single  SaturateOnIntegerOverflow=on
  w1 : Constant  Value=-g*Vehicle.Airframe.mass  OutDataTypeStr=single  SampleTime=Ts
  altitude_cmd : Outport
  Out Bus Element2 : Outport  Port=2  PortName=errors  Element=p
  Out Bus Element1 : Outport  Port=2  PortName=errors  Element=i
  Out Bus Element : Outport  Port=2  PortName=errors  Element=d
  wires:
  TakeoffOrControl_Switch1/1 -> Sum5/2
  PosZ/1 -> Sum2/1
  takeoff_flag/1 -> Terminator/1
  w1/1 -> Sum5/1, takeoff_gain1/1
  P_z/1 -> Out Bus Element2/1, Sum1/2
  Counter Free-Running/1 -> Compare To Constant/1
  Bus Selector1/2 -> D_z/1  "<dz>"
  Sum5/1 -> SaturationThrust1/1
  Bus Selector1/1 -> Sum2/2  "<Z>"
  D_z/1 -> Out Bus Element/1, Sum1/3  "dz"
  Sum1/1 -> TakeoffOrControl_Switch1/3
  Compare To Constant/1 -> TakeoffOrControl_Switch1/2, Discrete-Time Integrator2/2
  takeoff_gain1/1 -> TakeoffOrControl_Switch1/1
  states_estim/1 -> Bus Selector1/1
  Sum2/1 -> P_z/1, Add1/1  "pitch/roll error"
  SaturationThrust1/1 -> altitude_cmd/1
  Saturation1/1 -> Sum3/2, Sum1/1, Out Bus Element1/1
  Sum3/1 -> Delay1/1
  Delay1/1 -> antiWU_Gain1/1
  antiWU_Gain1/1 -> Add1/2
  mocap/1 -> Bus Selector/1
  I_z/1 -> Discrete-Time Integrator2/1
  Bus Selector/1 -> P_z/2  "<p_z>"
  Bus Selector/2 -> D_z/2  "<d_z>"
  Bus Selector/3 -> I_z/2  "<i_z>"
  Add1/1 -> I_z/1
  Discrete-Time Integrator2/1 -> Saturation1/1, Sum3/1

== system flightControlSystem/Flight Control System/Controller/thrustsToMotorCommands ==
  thrusts_refin : Inport
  MotorDirections : Gain  Gain=[1 -1 1 -1]
  Saturation5 : Saturate  UpperLimit=Vehicle.Motor.maxLimit  LowerLimit=Vehicle.Motor.minLimit
  ThrustToMotorCommand : Gain  Gain=-Vehicle.Motor.thrustToMotorCommand
  motors_cmdout : Outport
  wires:
  Saturation5/1 -> MotorDirections/1
  MotorDirections/1 -> motors_cmdout/1
  ThrustToMotorCommand/1 -> Saturation5/1
  thrusts_refin/1 -> ThrustToMotorCommand/1

== system flightControlSystem/Flight Control System/Crash Predictor Flags/Geofencing error ==
  Action Port : ActionPort  ActionPortLabel=if(u1 > 0)
  Constant : Constant  OutDataTypeStr=uint8
  Out1 : Outport
  wires:
  Constant/1 -> Out1/1

== system flightControlSystem/Flight Control System/Crash Predictor Flags/No optical flow  ==
  Action Port : ActionPort  ActionPortLabel=elseif( u3> 0)
  Constant : Constant  Value=69  OutDataTypeStr=uint8
  Out1 : Outport
  wires:
  Constant/1 -> Out1/1

== system flightControlSystem/Flight Control System/Crash Predictor Flags/Normal condition ==
  Action Port : ActionPort  ActionPortLabel=else
  Constant : Constant  Value=0  OutDataTypeStr=uint8
  Out1 : Outport
  wires:
  Constant/1 -> Out1/1

== system flightControlSystem/Flight Control System/Crash Predictor Flags/Ultrasound improper ==
  Action Port : ActionPort  ActionPortLabel=elseif(u4>0)
  Constant : Constant  Value=88  OutDataTypeStr=uint8
  Out1 : Outport
  wires:
  Constant/1 -> Out1/1

== system flightControlSystem/Flight Control System/Crash Predictor Flags/estimator//Optical flow error ==
  Action Port : ActionPort  ActionPortLabel=elseif(u2 > 0)
  Constant : Constant  Value=99  OutDataTypeStr=uint8
  Out1 : Outport
  wires:
  Constant/1 -> Out1/1

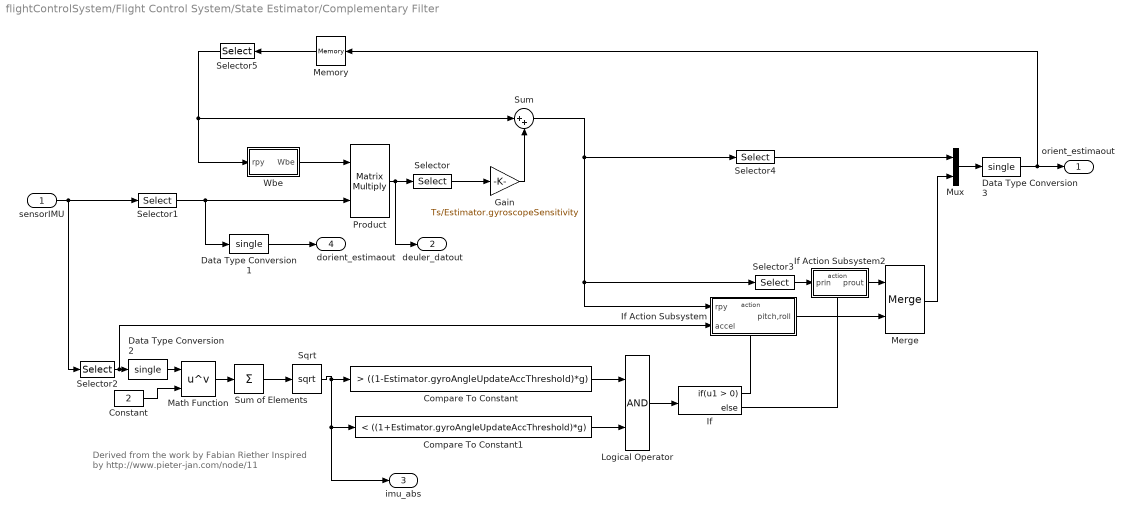
== system flightControlSystem/Flight Control System/State Estimator/Complementary Filter ==
  note: Derived from the work by Fabian Riether
      | Inspired by http://www.pieter-jan.com/node/11
  sensorIMU : Inport  OutDataTypeStr=single
  Compare To Constant : simulink/Logic and Bit Operations/Compare To Constant  relop=>  const=((1-Estimator.gyroAngleUpdateAccThreshold)*g)  OutDataTypeStr=boolean
  Compare To Constant1 : simulink/Logic and Bit Operations/Compare To Constant  relop=<  const=((1+Estimator.gyroAngleUpdateAccThreshold)*g)  OutDataTypeStr=boolean
  Constant : Constant  Value=2  OutDataTypeStr=single
  Data Type Conversion1 : DataTypeConversion  OutDataTypeStr=single
  Data Type Conversion2 : DataTypeConversion  OutDataTypeStr=single
  Data Type Conversion3 : DataTypeConversion  OutDataTypeStr=single
  Gain : Gain  Gain=Ts/Estimator.gyroscopeSensitivity
  If : If
  If Action Subsystem : Subsystem  TreatAsAtomicUnit=on
  If Action Subsystem2 : Subsystem  TreatAsAtomicUnit=on
  Logical Operator : Logic  AllPortsSameDT=off  OutDataTypeStr=fixdt(1,16)
  Math Function : Math  Operator=pow  SaturateOnIntegerOverflow=on
  Memory : Memory  InitialCondition=single(Estimator.complementaryFilterInit)  InheritSampleTime=on
  Merge : Merge
  Mux : Mux  Inputs=2
  Product : Product  Multiplication=Matrix(*)
  Selector : Selector  InputPortWidth=3  IndexOptions=Index vector (dialog)  Indices=[3 2 1]  OutputSizes=1
  Selector1 : Selector  InputPortWidth=6  IndexOptions=Index vector (dialog)  Indices=[4 5 6]  OutputSizes=1
  Selector2 : Selector  InputPortWidth=6  IndexOptions=Index vector (dialog)  Indices=[1 2 3]  OutputSizes=1
  Selector3 : Selector  InputPortWidth=3  IndexOptions=Index vector (dialog)  Indices=[2 1]  OutputSizes=1
  Selector4 : Selector  InputPortWidth=3  IndexOptions=Index vector (dialog)  Indices=[3]  OutputSizes=1
  Selector5 : Selector  InputPortWidth=3  IndexOptions=Index vector (dialog)  Indices=[3 2 1]  OutputSizes=1
  Sqrt : Sqrt  SaturateOnIntegerOverflow=on
  Sum : Sum  Inputs=|++
  Sum of Elements : Sum  Inputs=+
  Wbe : Subsystem
  orient_estimaout : Outport
  deuler_datout : Outport  Port=2
  imu_abs : Outport  Port=3  OutDataTypeStr=single
  dorient_estimaout : Outport  Port=4
  wires:
  sensorIMU/1 -> Selector1/1, Selector2/1
  Product/1 -> deuler_datout/1, Selector/1
  Wbe/1(Wbe) -> Product/1
  Selector/1 -> Gain/1
  Gain/1 -> Sum/2
  Memory/1 -> Selector5/1
  Sum of Elements/1 -> Sqrt/1
  Math Function/1 -> Sum of Elements/1
  Constant/1 -> Math Function/2
  Selector2/1 -> If Action Subsystem/2(accel), Data Type Conversion2/1
  Sqrt/1 -> imu_abs/1, Compare To Constant1/1, Compare To Constant/1
  Compare To Constant/1 -> Logical Operator/1
  Compare To Constant1/1 -> Logical Operator/2
  If Action Subsystem/1(pitch,roll) -> Merge/2
  Sum/1 -> If Action Subsystem/1(rpy), Selector3/1, Selector4/1
  Selector3/1 -> If Action Subsystem2/1(prin)
  Merge/1 -> Mux/2
  Mux/1 -> Data Type Conversion3/1
  If Action Subsystem2/1(prout) -> Merge/1
  If/2 -> If Action Subsystem2/Action
  Logical Operator/1 -> If/1
  If/1 -> If Action Subsystem/Action
  Selector1/1 -> Product/2, Data Type Conversion1/1
  Data Type Conversion2/1 -> Math Function/1
  Data Type Conversion3/1 -> Memory/1, orient_estimaout/1
  Selector5/1 -> Sum/1, Wbe/1(rpy)
  Data Type Conversion1/1 -> dorient_estimaout/1
  Selector4/1 -> Mux/1

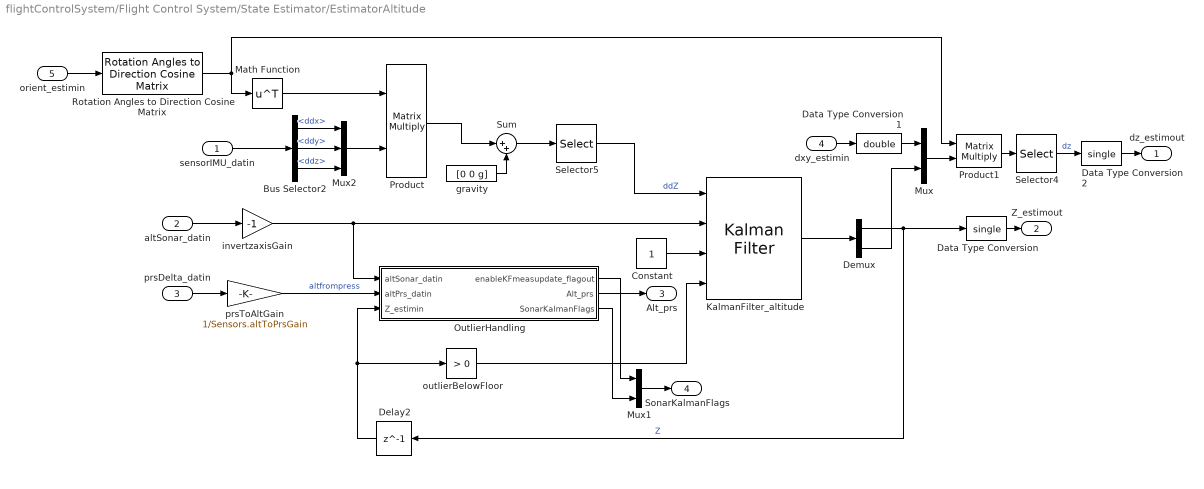
== system flightControlSystem/Flight Control System/State Estimator/EstimatorAltitude ==
  sensorIMU_datin : Inport
  altSonar_datin : Inport  Port=2
  prsDelta_datin : Inport  Port=3
  dxy_estimin : Inport  Port=4
  orient_estimin : Inport  Port=5
  Bus Selector2 : BusSelector  OutputSignals=ddx,ddy,ddz
  Constant : Constant
  Data Type Conversion : DataTypeConversion  OutDataTypeStr=single  SaturateOnIntegerOverflow=on
  Data Type Conversion1 : DataTypeConversion  OutDataTypeStr=double  SaturateOnIntegerOverflow=on
  Data Type Conversion2 : DataTypeConversion  OutDataTypeStr=single  SaturateOnIntegerOverflow=on
  Delay2 : Delay  DelayLength=1  InitialCondition=0
  Demux : Demux  Outputs=2
  KalmanFilter_altitude : ctrlSharedLib/Kalman Filter  TimeDomain=Discrete-Time  UseCurrentEstimator=on  ModelSource=Individual A, B, C, D matrices  ModelSourceVariable=sys  A=[1 Ts; 0 1]  B=[0;Ts]  C=[1 0]  D=[0]  NumberOfStates=2  NumberOfInputs=2  NumberOfOutputs=2  InitialEstimateSource=Dialog  X0=[init.posNED(3) 0]  P0=10  UseK=off  UseGH=on  NumberOfProcessNoiseInputs=2  G=Estimator.alt.kf.G  TimeInvariantG=on  H=Estimator.alt.kf.H  TimeInvariantH=on  Q=Estimator.alt.kf.Q  TimeInvariantQ=on  R=Estimator.alt.kf.R  TimeInvariantR=on  N=Estimator.alt.kf.N  TimeInvariantN=on  AddInputPort=on  AddEnablePort=on  ExternalReset=Level hold  OutputEstimatedY=off  OutputP=off  Ts=-1
  Math Function : Math  Operator=transpose  SaturateOnIntegerOverflow=on
  Mux : Mux  Inputs=2
  Mux1 : Mux  Inputs=2
  Mux2 : Mux  Inputs=3
  OutlierHandling : Subsystem
  Product : Product  Multiplication=Matrix(*)
  Product1 : Product  Multiplication=Matrix(*)
  Rotation Angles to Direction Cosine Matrix : sharedtransform/Rotation Angles to Direction Cosine Matrix  rotationOrder=ZYX  aMode=aMode
  Selector4 : Selector  InputPortWidth=3  IndexOptions=Index vector (dialog)  Indices=[3]  OutputSizes=1
  Selector5 : Selector  InputPortWidth=3  IndexOptions=Index vector (dialog)  Indices=[3]  OutputSizes=1
  Sum : Sum  Inputs=|++
  gravity : Constant  Value=[0 0 g]
  invertzaxisGain : Gain  Gain=-1  ParamDataTypeStr=single  OutDataTypeStr=double
  outlierBelowFloor : simulink/Logic and Bit Operations/Compare To Constant  relop=>  const=0  OutDataTypeStr=boolean
  prsToAltGain : Gain  Gain=1/Sensors.altToPrsGain
  dz_estimout : Outport
  Z_estimout : Outport  Port=2
  Alt_prs : Outport  Port=3
  SonarKalmanFlags : Outport  Port=4
  wires:
  Mux2/1 -> Product/2
  sensorIMU_datin/1 -> Bus Selector2/1
  Bus Selector2/3 -> Mux2/3  "<ddz>"
  Bus Selector2/2 -> Mux2/2  "<ddy>"
  Bus Selector2/1 -> Mux2/1  "<ddx>"
  Product1/1 -> Selector4/1
  dxy_estimin/1 -> Data Type Conversion1/1
  Delay2/1 -> OutlierHandling/3(Z_estimin), outlierBelowFloor/1
  prsToAltGain/1 -> OutlierHandling/2(altPrs_datin)  "altfrompress"
  prsDelta_datin/1 -> prsToAltGain/1
  outlierBelowFloor/1 -> KalmanFilter_altitude/4
  Demux/2 -> Mux/2
  Selector4/1 -> Data Type Conversion2/1  "dz"
  Demux/1 -> Data Type Conversion/1, Delay2/1  "Z"
  Selector5/1 -> KalmanFilter_altitude/1  "ddZ"
  Mux/1 -> Product1/2
  KalmanFilter_altitude/1 -> Demux/1
  Sum/1 -> Selector5/1
  gravity/1 -> Sum/2
  Product/1 -> Sum/1
  altSonar_datin/1 -> invertzaxisGain/1
  orient_estimin/1 -> Rotation Angles to Direction Cosine Matrix/1
  Data Type Conversion/1 -> Z_estimout/1
  Data Type Conversion1/1 -> Mux/1
  Math Function/1 -> Product/1
  invertzaxisGain/1 -> KalmanFilter_altitude/2, OutlierHandling/1(altSonar_datin)
  Data Type Conversion2/1 -> dz_estimout/1
  OutlierHandling/1(enableKFmeasupdate_flagout) -> Mux1/1
  Rotation Angles to Direction Cosine Matrix/1 -> Math Function/1, Product1/1
  OutlierHandling/2(Alt_prs) -> Alt_prs/1
  OutlierHandling/3(SonarKalmanFlags) -> Mux1/2
  Mux1/1 -> SonarKalmanFlags/1
  Constant/1 -> KalmanFilter_altitude/3

== system flightControlSystem/Flight Control System/State Estimator/EstimatorXYPosition ==
  opticalFlow_datin : Inport
  controlModePosVSOrient_flagin : Inport  Port=2
  sensorIMU_datin : Inport  Port=3
  Z_estimin : Inport  Port=4
  dz_estimin : Inport  Port=5
  orient_estimin : Inport  Port=6
  EstimatorVelocity : Subsystem
  EstimatorXYPosition : Subsystem
  XY_estimout : Outport
  dxy_estimout : Outport  Port=2
  flag_track : Outport  Port=3
  wires:
  EstimatorXYPosition/1(XY_estimout) -> XY_estimout/1
  dz_estimin/1 -> EstimatorXYPosition/4(dz_estimin)
  controlModePosVSOrient_flagin/1 -> EstimatorXYPosition/3(controlModePosVSOrient_flagin)
  Z_estimin/1 -> EstimatorVelocity/2(Z_estimin)
  sensorIMU_datin/1 -> EstimatorVelocity/3(sensorIMU_datin)
  opticalFlow_datin/1 -> EstimatorVelocity/1(opticalFlow_datin)
  EstimatorVelocity/1(dxy_estimout) -> dxy_estimout/1, EstimatorXYPosition/1(dxy_estimin)
  orient_estimin/1 -> EstimatorVelocity/4(orient_estimin), EstimatorXYPosition/2(orient_estimin)
  EstimatorVelocity/2(flag_track) -> flag_track/1

== system flightControlSystem/Flight Control System/State Estimator/SensorPreprocessing ==
  note: IMU
  sensordata_datin : Inport
  sensorCalibration_datin : Inport  Port=2
  Assuming that calib was done level! : Bias  Bias=[0 0 +g 0 0 0]
  Bus Creator3 : BusCreator  Inputs=6
  Bus Selector : BusSelector  OutputSignals=ddx,ddy,ddz,p,q,r
  Bus Selector1 : BusSelector  OutputSignals=altitude_sonar,prs
  Bus Selector2 : BusSelector  OutputSignals=HAL_acc_SI,HAL_gyro_SI,HAL_ultrasound_SI,HAL_pressure_SI,HAL_vbat_SI
  Bus Selector3 : BusSelector  OutputSignals=HALSensors
  Data Type Conversion : DataTypeConversion
  Demux1 : Demux  Outputs=3
  Demux2 : Demux  Outputs=3
  FIR_IMUaccel : DiscreteFir  Coefficients=Estimator.IMU.filterAccel.Coefficients
  IIR_IMUgyro_r : DiscreteFilter  Numerator=Estimator.IMU.filterGyroNum  Denominator=Estimator.IMU.filterGyroDen
  Mux1 : Mux  Inputs=6
  Select Accel : Selector  InputPortWidth=6  IndexOptions=Index vector (dialog)  Indices=[1 2 3]  OutputSizes=1
  Select pqr : Selector  InputPortWidth=6  IndexOptions=Index vector (dialog)  Indices=[4 5 6]  OutputSizes=1
  Selector2 : Selector  InputPortWidth=8  IndexOptions=Index vector (dialog)  Indices=[1:6]  OutputSizes=1
  Selector4 : Selector  InputPortWidth=8  IndexOptions=Index vector (dialog)  Indices=[7]  OutputSizes=1
  Sum1 : Sum  Inputs=|+-
  Sum2 : Sum  Inputs=-+|
  inverseIMU_gain : Gain  Gain=Estimator.inverseIMUGain  ParamDataTypeStr=single  OutDataTypeStr=single
  sensordata_group : Subsystem
  sensorIMU_datout : Outport
  altSonar_datout : Outport  Port=2
  prsDelta_datout : Outport  Port=3
  wires:
  Select pqr/1 -> Demux2/1
  Assuming that calib was done level!/1 -> Sum1/2
  Mux1/1 -> Sum1/1
  Sum2/1 -> prsDelta_datout/1
  Bus Selector1/2 -> Sum2/2  "<prs>"
  Selector4/1 -> Sum2/1
  Bus Selector1/1 -> altSonar_datout/1  "<altitude_sonar>"
  Bus Selector/6 -> Mux1/6  "<r>"
  Bus Selector/5 -> Mux1/5  "<q>"
  Bus Selector/4 -> Mux1/4  "<p>"
  Bus Selector/3 -> Mux1/3  "<ddz>"
  Bus Selector/2 -> Mux1/2  "<ddy>"
  Bus Selector/1 -> Mux1/1  "<ddx>"
  sensorCalibration_datin/1 -> Data Type Conversion/1
  IIR_IMUgyro_r/1 -> Bus Creator3/6  "r"
  Demux2/3 -> IIR_IMUgyro_r/1  "r"
  FIR_IMUaccel/1 -> Demux1/1
  Select Accel/1 -> FIR_IMUaccel/1
  inverseIMU_gain/1 -> Select Accel/1, Select pqr/1
  Demux2/2 -> Bus Creator3/5  "q"
  Demux2/1 -> Bus Creator3/4  "p"
  Selector2/1 -> Assuming that calib was done level!/1
  Sum1/1 -> inverseIMU_gain/1
  Demux1/3 -> Bus Creator3/3  "ddz"
  Demux1/2 -> Bus Creator3/2  "ddy"
  Demux1/1 -> Bus Creator3/1  "ddx"
  Bus Creator3/1 -> sensorIMU_datout/1
  Data Type Conversion/1 -> Selector2/1, Selector4/1
  Bus Selector2/2 -> sensordata_group/2(HAL_gyro_SI)  "<HAL_gyro_SI>"
  Bus Selector2/4 -> sensordata_group/4(HAL_pressure_SI)  "<HAL_pressure_SI>"
  Bus Selector2/5 -> sensordata_group/5(HAL_vbat_SI)  "<HAL_vbat_SI>"
  Bus Selector2/3 -> sensordata_group/3(HAL_ultrasound_SI)  "<HAL_ultrasound_SI>"
  Bus Selector3/1 -> Bus Selector2/1  "<HALSensors>"
  sensordata_group/1(sensordata_datin) -> Bus Selector1/1, Bus Selector/1
  sensordata_datin/1 -> Bus Selector3/1
  Bus Selector2/1 -> sensordata_group/1(HAL_acc_SI)  "<HAL_acc_SI>"

== system flightControlSystem/Flight Control System/State Estimator/Complementary Filter/If Action Subsystem ==
  rpy : Inport
  accel : Inport  Port=2
  Action Port : ActionPort  ActionPortLabel=if(u1 > 0)
  Demux : Demux  Outputs=3
  Demux1 : Demux  Outputs=3
  Divide : Product  Inputs=*/
  Gain : Gain  Gain=1-Estimator.gyroAngleUpdateAccWeight
  Gain1 : Gain  Gain=Estimator.gyroAngleUpdateAccWeight
  Gain2 : Gain  Gain=1/g
  Gain3 : Gain  Gain=Estimator.gyroAngleUpdateAccWeight
  Gain4 : Gain  Gain=1-Estimator.gyroAngleUpdateAccWeight
  Mux : Mux  Inputs=2
  Sum : Sum  Inputs=|++
  Sum1 : Sum  Inputs=|++
  Terminator1 : Terminator
  Trigonometric Function : Trigonometry  Operator=atan
  Trigonometric Function1 : Trigonometry  Operator=asin
  pitch,roll : Outport
  wires:
  accel/1 -> Demux/1
  Demux/2 -> Divide/1
  Demux/3 -> Divide/2
  Divide/1 -> Trigonometric Function/1
  Gain/1 -> Sum/1
  Trigonometric Function/1 -> Gain1/1
  Mux/1 -> pitch,roll/1
  Gain2/1 -> Trigonometric Function1/1
  Trigonometric Function1/1 -> Gain3/1
  Gain4/1 -> Sum1/1
  Gain3/1 -> Sum1/2
  Sum1/1 -> Mux/1
  Sum/1 -> Mux/2
  rpy/1 -> Demux1/1
  Demux1/1 -> Gain/1
  Demux1/2 -> Gain4/1
  Demux/1 -> Gain2/1
  Demux1/3 -> Terminator1/1
  Gain1/1 -> Sum/2

== system flightControlSystem/Flight Control System/State Estimator/Complementary Filter/If Action Subsystem2 ==
  prin : Inport
  Action Port : ActionPort  ActionPortLabel=else
  prout : Outport
  wires:
  prin/1 -> prout/1

== system flightControlSystem/Flight Control System/State Estimator/Complementary Filter/Wbe ==
  rpy : Inport  OutDataTypeStr=single
  Constant : Constant  Value=single(0)
  Create 3x3 Matrix : sharedutil/Create 3x3 Matrix  aMode=aMode
  Divide : Product  Inputs=*/
  Gain : Gain  Gain=-1
  Product{1..4} (4 alike) : Product
  Selector : Selector  InputPortWidth=3  IndexOptions=Index vector (dialog)  Indices=[1]  OutputSizes=1
  Selector1 : Selector  InputPortWidth=3  IndexOptions=Index vector (dialog)  Indices=[1]  OutputSizes=1
  Selector2 : Selector  InputPortWidth=3  IndexOptions=Index vector (dialog)  Indices=[2]  OutputSizes=1
  Selector3 : Selector  InputPortWidth=3  IndexOptions=Index vector (dialog)  Indices=[2]  OutputSizes=1
  Trigonometric Function : Trigonometry  Operator=sincos
  Wbe : Outport
  wires:
  Create 3x3 Matrix/1 -> Divide/1
  Product3/1 -> Create 3x3 Matrix/8
  Trigonometric Function/2 -> Selector1/1, Selector2/1
  Selector3/1 -> Product4/2, Product3/2
  Selector1/1 -> Product4/1, Product1/1, Create 3x3 Matrix/3
  Trigonometric Function/1 -> Selector3/1, Selector/1
  Product1/1 -> Create 3x3 Matrix/5
  Product2/1 -> Create 3x3 Matrix/6
  Selector2/1 -> Divide/2, Create 3x3 Matrix/7, Product2/1, Product1/2
  Gain/1 -> Product2/2
  Product4/1 -> Create 3x3 Matrix/9
  Constant/1 -> Create 3x3 Matrix/4, Create 3x3 Matrix/1
  Divide/1 -> Wbe/1
  rpy/1 -> Trigonometric Function/1
  Selector/1 -> Product3/1, Gain/1, Create 3x3 Matrix/2
